simulink model "Es5_sim"  (R2017b)
settings: Solver=VariableStepAuto  StartTime=0.0  StopTime=10.0  RelTol=1e-3
values from neighbouring files (symbols this model uses):
  x0 = [-1.5 -1.5]    [Es5.m]
libraries: simulink x1
settings Model: Creator=claudio  LastModifiedBy=claudio

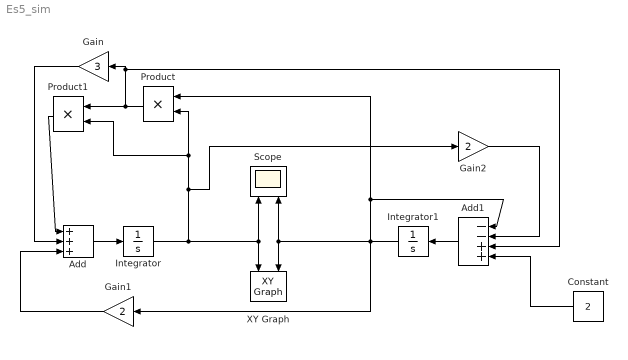
== system Es5_sim ==
  Add : Sum  Inputs=+++
  Add1 : Sum  Inputs=--++
  Constant : Constant  Value=2
  Gain : Gain  Gain=3
  Gain1 : Gain  Gain=2
  Gain2 : Gain  Gain=2
  Integrator : Integrator  InitialCondition=x0(1)
  Integrator1 : Integrator  InitialCondition=x0(2)
  Product : Product
  Product1 : Product
  Scope : Scope  NumInputPorts=2
  XY Graph : simulink/Sinks/XY Graph  xmin=-5  xmax=5  ymin=-5  ymax=5  st=-1
  wires:
  Add/1 -> Integrator/1
  Integrator/1 -> Scope/1, XY Graph/1, Gain2/1, Product1/2, Product/2
  Integrator1/1 -> Scope/2, XY Graph/2, Gain1/1, Add1/1, Product/1
  Product/1 -> Add1/3, Gain/1, Product1/1
  Product1/1 -> Add/1
  Gain/1 -> Add/2
  Gain1/1 -> Add/3
  Add1/1 -> Integrator1/1
  Gain2/1 -> Add1/2
  Constant/1 -> Add1/4
